simulink model "robot_tfModel"  (R2020b)
settings: Solver=FixedStepDiscrete  StartTime=0.0  StopTime=10  FixedStep=1e-3  MaxStep=1e-3  RelTol=1e-3
undefined symbols (not defined in the file or in its folder): a, b, c, d
libraries: cstblocks x3
settings Model: Creator=User  LastModifiedBy=root

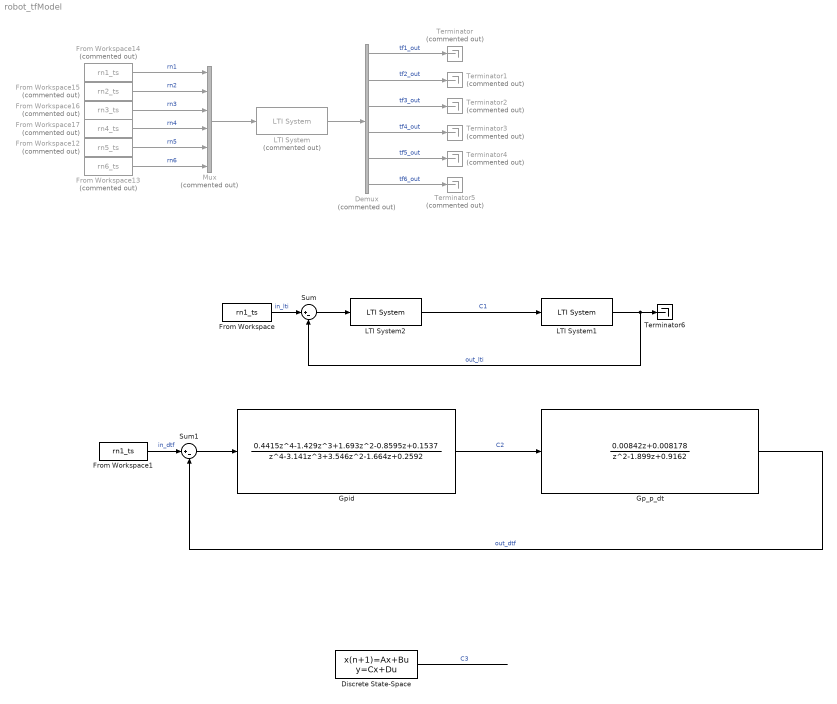
== system robot_tfModel ==
  Demux : Demux  Commented=on  Outputs=6
  Discrete State-Space : DiscreteStateSpace  A=a  B=b  C=c  D=d  SampleTime=1e-3
  From Workspace : FromWorkspace  VariableName=rn1_ts  Interpolate=off  OutputAfterFinalValue=Holding final value
  From Workspace1 : FromWorkspace  VariableName=rn1_ts  Interpolate=off  OutputAfterFinalValue=Holding final value
  From Workspace12 : FromWorkspace  Commented=on  VariableName=rn5_ts
  From Workspace13 : FromWorkspace  Commented=on  VariableName=rn6_ts
  From Workspace14 : FromWorkspace  Commented=on  VariableName=rn1_ts  SampleTime=1e-3
  From Workspace15 : FromWorkspace  Commented=on  VariableName=rn2_ts
  From Workspace16 : FromWorkspace  Commented=on  VariableName=rn3_ts
  From Workspace17 : FromWorkspace  Commented=on  VariableName=rn4_ts
  Gp_p_dt : DiscreteTransferFcn  Numerator="[0 0.00842  0.008178]"  Denominator=[1 -1.899 0.9162]
  Gpid : DiscreteTransferFcn  Numerator=[0.4415 -1.429 1.693 -0.8595 0.1537]  Denominator=[1 -3.141 3.546 -1.664 0.2592]  a0EqualsOne=on
  LTI System : cstblocks/LTI System  Commented=on  sys=dtf  IC=[]
  LTI System1 : cstblocks/LTI System  sys=Gp_p_dt  IC=[]
  LTI System2 : cstblocks/LTI System  sys=Gpid_dt  IC=[]
  Mux : Mux  Commented=on  Inputs=6
  Sum : Sum  Inputs=|+-
  Sum1 : Sum  Inputs=|+-
  Terminator{,1..5} (6 alike) : Terminator  Commented=on
  Terminator6 : Terminator
  wires:
  Mux/1 -> LTI System/1
  LTI System/1 -> Demux/1
  Demux/1 -> Terminator/1  "tf1_out"
  Demux/2 -> Terminator1/1  "tf2_out"
  Demux/3 -> Terminator2/1  "tf3_out"
  Demux/4 -> Terminator3/1  "tf4_out"
  Demux/5 -> Terminator4/1  "tf5_out"
  Demux/6 -> Terminator5/1  "tf6_out"
  From Workspace15/1 -> Mux/2  "rn2"
  From Workspace12/1 -> Mux/5  "rn5"
  From Workspace17/1 -> Mux/4  "rn4"
  From Workspace13/1 -> Mux/6  "rn6"
  From Workspace14/1 -> Mux/1  "rn1"
  From Workspace16/1 -> Mux/3  "rn3"
  LTI System1/1 -> Sum/2, Terminator6/1  "out_lti"
  LTI System2/1 -> LTI System1/1  "C1"
  Sum/1 -> LTI System2/1
  Gpid/1 -> Gp_p_dt/1  "C2"
  Sum1/1 -> Gpid/1
  Gp_p_dt/1 -> Sum1/2  "out_dtf"
  From Workspace1/1 -> Sum1/1  "in_dtf"
  Discrete State-Space/1 -> ?  "C3"
  From Workspace/1 -> Sum/1  "in_lti"
